simulink model "decodeIdString"  (R2019b)
settings: Solver=VariableStepAuto  StartTime=0.0  StopTime=10.0  RelTol=1e-3
settings Model: Creator=y0n  LastModifiedBy=y0n

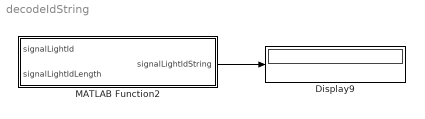
== system decodeIdString ==
  Display9 : Display
  MATLAB Function2 : MATLAB Function  TreatAsAtomicUnit=on  SystemSampleTime=0.001
  wires:
  MATLAB Function2/1(signalLightIdString) -> Display9/1

== matlab function decodeIdString/MATLAB Function2 ==
  data: signalLightId input uint8 size=[1 50]; signalLightIdString output string; signalLightIdLength input
function signalLightIdString = fcn(signalLightId, signalLightIdLength)

signalLightIdString = string(char(signalLightId));
